simulink model "ADRC"  (R2023a)
settings: Solver=FixedStepAuto  StartTime=0.0  StopTime=10  FixedStep=0.00001  MaxStep=0.001  RelTol=1e-3
values from neighbouring files (symbols this model uses):
  J = 0.00027    [untitled.m]
  kp = W/N    (= 0.17)    [untitled.m]
undefined symbols (not defined in the file or in its folder): alph1, alph2, alph3, b0, kd
libraries: slctrl_adaptive x1
settings Model: Creator=ZJX  LastModifiedBy=ZJX
settings OptimizationCC: BlockReduction=off  DefaultParameterBehavior=Inlined  EnhancedBackFolding=on  PassReuseOutputArgsAs=Individual arguments  ZeroExternalMemoryAtStartup=off  ZeroInternalMemoryAtStartup=off  OptimizeBlockOrder=speed  DifferentSizesBufferReuse=on  OptimizationCustomize=off  EfficientTunableParamExpr=on
settings DebuggingCC: ParameterTunabilityLossMsg=error
settings SFSimCC: MATLABDynamicMemAlloc=off
settings RTWCC: Description=Embedded Coder  SystemTargetFile=ert.tlc  TemplateMakefile=ert_default_tmf  Toolchain=MinGW64 | CMake/gmake (64-bit Windows)  BuildConfiguration=Release
settings CodeAppCC: ForceParamTrailComments=on  IgnoreCustomStorageClasses=off  OperatorAnnotations=on  SimulinkDataObjDesc=on  SFDataObjDesc=on  InsertBlockDesc=on
settings ERTTargetCC: TargetLangStandard=C99 (ISO)  GenerateSampleERTMain=on  InlinedParameterPlacement=NonHierarchical  ERTCustomFileTemplate=example_file_process.tlc

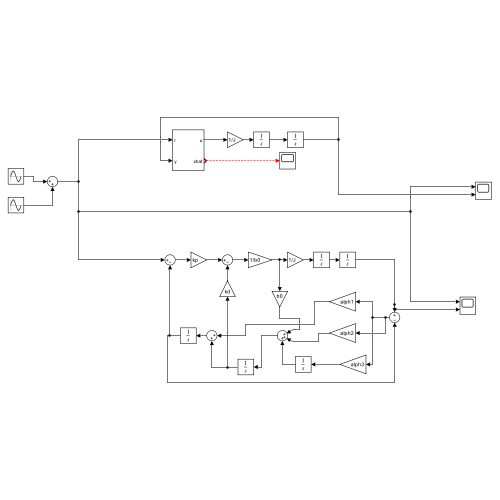
[thumbnail: Simulink's stored preview of the top-level diagram]
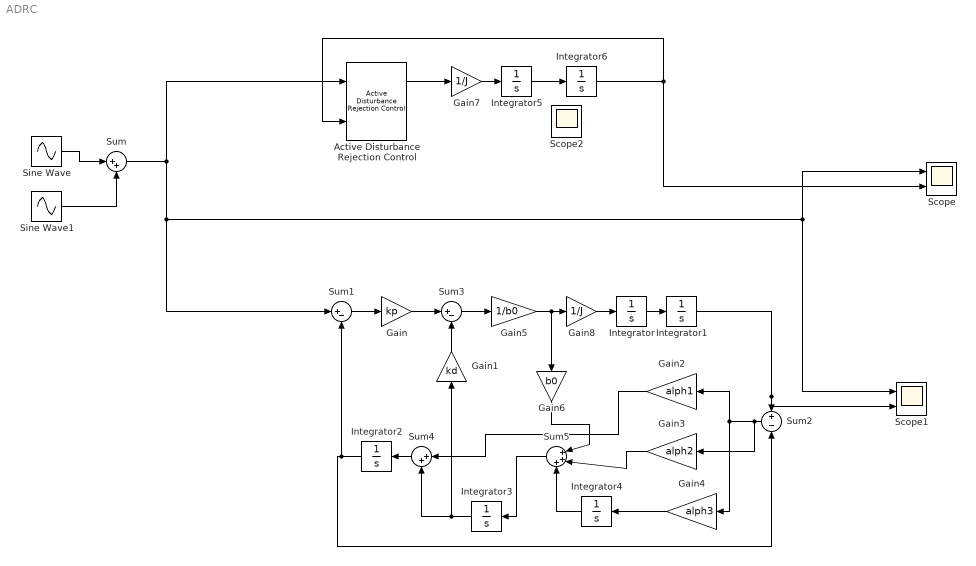
== system ADRC ==
  Active Disturbance Rejection Control : slctrl_adaptive/Active Disturbance Rejection Control  time_domain=continuous-time  Ts=0.00001  model_type=second-order  b0=1/J  wc=400  wo=1200  x0=0  ulim_checkbox=off  umax=inf  umin=-inf  xhat_checkbox=on
      settings: LibrarySourceBlock=slctrlblks/Adaptive Control/Active Disturbance Rejection Control
  Gain : Gain  Gain=kp
  Gain1 : Gain  Gain=kd
  Gain2 : Gain  Gain=alph1
  Gain3 : Gain  Gain=alph2
  Gain4 : Gain  Gain=alph3
  Gain5 : Gain  Gain=1/b0
  Gain6 : Gain  Gain=b0
  Gain7 : Gain  Gain=1/J
  Gain8 : Gain  Gain=1/J
  Integrator{,1..6} (7 alike) : Integrator
  Scope : Scope  NumInputPorts=2
  Scope1 : Scope  NumInputPorts=2
  Scope2 : Scope
  Sine Wave : Sin  Frequency=50  SampleTime=0
  Sine Wave1 : Sin  Amplitude=0.05  Frequency=500  SampleTime=0
  Sum : Sum  Inputs=|++
  Sum1 : Sum  Inputs=|+-
  Sum2 : Sum  Inputs=+|-
  Sum3 : Sum  Inputs=|+-
  Sum4 : Sum  Inputs=|++
  Sum5 : Sum  Inputs=|+++
  wires:
  Integrator5/1 -> Integrator6/1
  Sine Wave/1 -> Sum/1
  Sine Wave1/1 -> Sum/2
  Sum1/1 -> Gain/1
  Integrator2/1 -> Sum1/2, Sum2/2
  Integrator1/1 -> Sum2/1, Scope1/2
  Gain/1 -> Sum3/1
  Gain1/1 -> Sum3/2
  Integrator3/1 -> Sum4/2, Gain1/1
  Sum4/1 -> Integrator2/1
  Sum5/1 -> Integrator3/1
  Gain4/1 -> Integrator4/1
  Integrator4/1 -> Sum5/3
  Gain3/1 -> Sum5/2
  Sum2/1 -> Gain2/1, Gain4/1, Gain3/1
  Gain5/1 -> Gain8/1, Gain6/1
  Sum3/1 -> Gain5/1
  Gain6/1 -> Sum5/1
  Gain2/1 -> Sum4/1
  ? -> Scope2/1
  Sum/1 -> Sum1/1, Scope1/1, Scope/1, Active Disturbance Rejection Control/1
  Active Disturbance Rejection Control/1 -> Gain7/1
  Gain8/1 -> Integrator/1
  Integrator/1 -> Integrator1/1
  Gain7/1 -> Integrator5/1
  Integrator6/1 -> Scope/2, Active Disturbance Rejection Control/2
